simulink model "Online_Ordering_System_Component_Architecture"  (R2025a)
settings: Solver=VariableStepDiscrete  StartTime=0.0  StopTime=10.0  MaxStep=1  RelTol=1e-3
(part 1 of 2)
settings Model: Creator=OdaNobuyuki  LastModifiedBy=annic

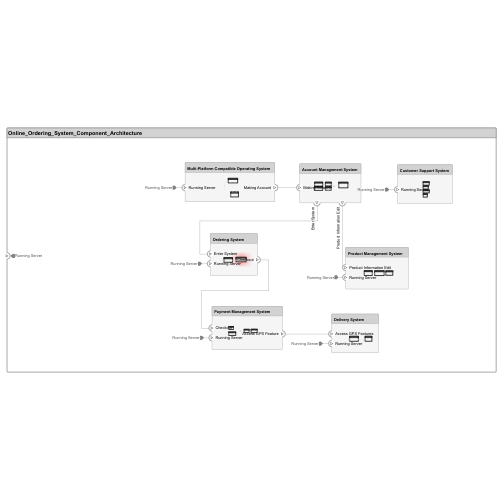
[thumbnail: Simulink's stored preview of the top-level diagram]
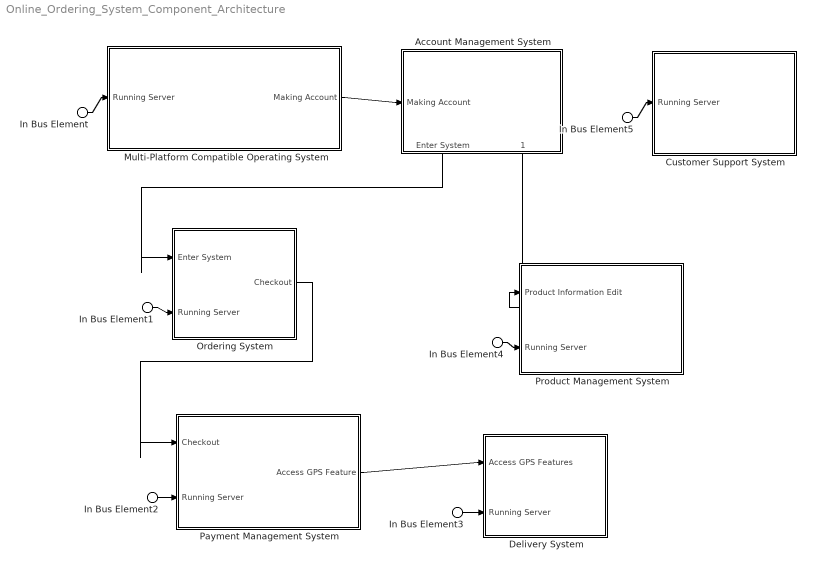
== system Online_Ordering_System_Component_Architecture ==
  In Bus Element{,1..5} (6 alike) : Inport  PortName=Running Server
  Account Management System : Subsystem
      settings: PortSchema="{\"entries\":[{\"content\":{\"headerSize\":26,\"margin\":15,\"minimumSpacing\":25,\"sides\":[{\"content\":{\"connectorIds\":[\"In1\"]},\"type\":\"ConnectorPlacement.EquallySpacedRectSide\",\"uuid\":\"d2ebed04-42f4-4bd6-aa56-c214d37abe86\"},{\"content\":{\"side\":\"RIGHT\"},\"type\":\"ConnectorPlacement.EquallySpacedRectSide\",\"uuid\":\"0a328130-2da5-4535-b8fd-dee261bd04a3\"},{\"content\":{\"side\":\"TOP\"},\"type\":\"ConnectorPlacement.EquallySpacedRectSide\",\"uuid\":\"410ea5eb-e20b-4523-bb7e-a86253749ceb\"},{\"content\":{\"connectorIds\":[\"Out2\",\"Out1\"],\"side\":\"BOTTOM\"},\"type\":\"ConnectorPlacement.EquallySpacedRectSide\",\"uuid\":\"972444bc-2579-4da8-b46a-55dab0c65c8e\"}]},\"type\":\"ConnectorPlacement.EquallySpacedConnector\",\"uuid\":\"5600d62f-d466-4629-981b-50f24b9b11a3\"}],\"packageUris\":[\"http://schema.mathworks.com/mf0/Connector/R2020b\"],\"version\":\"1.0\"}"
  "Customer Support System " : Subsystem
      settings: PortSchema="{\"entries\":[{\"content\":{\"headerSize\":26,\"margin\":15,\"minimumSpacing\":25,\"sides\":[{\"content\":{\"connectorIds\":[\"In1\"]},\"type\":\"ConnectorPlacement.EquallySpacedRectSide\",\"uuid\":\"fb288abb-f281-4c09-9d66-d398814e9f3f\"},{\"content\":{\"side\":\"RIGHT\"},\"type\":\"ConnectorPlacement.EquallySpacedRectSide\",\"uuid\":\"124df975-d2be-4c45-a02a-2f8c5952e2b0\"},{\"content\":{\"side\":\"TOP\"},\"type\":\"ConnectorPlacement.EquallySpacedRectSide\",\"uuid\":\"1b6fa379-ab8e-486c-bf17-64ebd19504fb\"}]},\"type\":\"ConnectorPlacement.EquallySpacedConnector\",\"uuid\":\"3496844b-ca8f-4528-b99e-6963a01fd8b6\"}],\"packageUris\":[\"http://schema.mathworks.com/mf0/Connector/R2020b\"],\"version\":\"1.0\"}"
  Delivery System : Subsystem
      settings: PortSchema="{\"entries\":[{\"content\":{\"headerSize\":26,\"margin\":15,\"minimumSpacing\":25,\"sides\":[{\"content\":{\"connectorIds\":[\"In1\",\"In2\"]},\"type\":\"ConnectorPlacement.EquallySpacedRectSide\",\"uuid\":\"d2ebed04-42f4-4bd6-aa56-c214d37abe86\"},{\"content\":{\"side\":\"RIGHT\"},\"type\":\"ConnectorPlacement.EquallySpacedRectSide\",\"uuid\":\"0a328130-2da5-4535-b8fd-dee261bd04a3\"},{\"content\":{\"side\":\"TOP\"},\"type\":\"ConnectorPlacement.EquallySpacedRectSide\",\"uuid\":\"410ea5eb-e20b-4523-bb7e-a86253749ceb\"}]},\"type\":\"ConnectorPlacement.EquallySpacedConnector\",\"uuid\":\"5600d62f-d466-4629-981b-50f24b9b11a3\"}],\"packageUris\":[\"http://schema.mathworks.com/mf0/Connector/R2020b\"],\"version\":\"1.0\"}"
  "Multi-Platform Compatible Operating System " : Subsystem
      settings: PortSchema="{\"entries\":[{\"content\":{\"headerSize\":26,\"margin\":15,\"minimumSpacing\":25,\"sides\":[{\"content\":{\"connectorIds\":[\"In1\"]},\"type\":\"ConnectorPlacement.EquallySpacedRectSide\",\"uuid\":\"fb288abb-f281-4c09-9d66-d398814e9f3f\"},{\"content\":{\"connectorIds\":[\"Out1\"],\"side\":\"RIGHT\"},\"type\":\"ConnectorPlacement.EquallySpacedRectSide\",\"uuid\":\"124df975-d2be-4c45-a02a-2f8c5952e2b0\"},{\"content\":{\"side\":\"TOP\"},\"type\":\"ConnectorPlacement.EquallySpacedRectSide\",\"uuid\":\"1b6fa379-ab8e-486c-bf17-64ebd19504fb\"}]},\"type\":\"ConnectorPlacement.EquallySpacedConnector\",\"uuid\":\"3496844b-ca8f-4528-b99e-6963a01fd8b6\"}],\"packageUris\":[\"http://schema.mathworks.com/mf0/Connector/R2020b\"],\"version\":\"1.0\"}"
  Ordering System : Subsystem
      settings: PortSchema="{\"entries\":[{\"content\":{\"headerSize\":26,\"margin\":15,\"minimumSpacing\":25,\"sides\":[{\"content\":{\"connectorIds\":[\"In1\",\"In2\"]},\"type\":\"ConnectorPlacement.EquallySpacedRectSide\",\"uuid\":\"fb288abb-f281-4c09-9d66-d398814e9f3f\"},{\"content\":{\"connectorIds\":[\"Out1\"],\"side\":\"RIGHT\"},\"type\":\"ConnectorPlacement.EquallySpacedRectSide\",\"uuid\":\"124df975-d2be-4c45-a02a-2f8c5952e2b0\"},{\"content\":{\"side\":\"TOP\"},\"type\":\"ConnectorPlacement.EquallySpacedRectSide\",\"uuid\":\"1b6fa379-ab8e-486c-bf17-64ebd19504fb\"}]},\"type\":\"ConnectorPlacement.EquallySpacedConnector\",\"uuid\":\"3496844b-ca8f-4528-b99e-6963a01fd8b6\"}],\"packageUris\":[\"http://schema.mathworks.com/mf0/Connector/R2020b\"],\"version\":\"1.0\"}"
  "Payment Management System " : Subsystem
      settings: PortSchema="{\"entries\":[{\"content\":{\"headerSize\":26,\"margin\":15,\"minimumSpacing\":25,\"sides\":[{\"content\":{\"connectorIds\":[\"In1\",\"In2\"]},\"type\":\"ConnectorPlacement.EquallySpacedRectSide\",\"uuid\":\"c87fdfc5-e8df-459e-b997-08543d0df41e\"},{\"content\":{\"connectorIds\":[\"Out1\"],\"side\":\"RIGHT\"},\"type\":\"ConnectorPlacement.EquallySpacedRectSide\",\"uuid\":\"2c60bf56-1d16-41c9-95da-6f31ce1e2453\"},{\"content\":{\"side\":\"TOP\"},\"type\":\"ConnectorPlacement.EquallySpacedRectSide\",\"uuid\":\"3204d3ae-6da8-4da9-829b-7d815393aaef\"}]},\"type\":\"ConnectorPlacement.EquallySpacedConnector\",\"uuid\":\"82e413f9-6f35-4bf6-9ebc-f322256f270e\"}],\"packageUris\":[\"http://schema.mathworks.com/mf0/Connector/R2020b\"],\"version\":\"1.0\"}"
  Product Management System : Subsystem
      settings: PortSchema="{\"entries\":[{\"content\":{\"headerSize\":26,\"margin\":15,\"minimumSpacing\":25,\"sides\":[{\"content\":{\"connectorIds\":[\"In1\",\"In2\"]},\"type\":\"ConnectorPlacement.EquallySpacedRectSide\",\"uuid\":\"fb288abb-f281-4c09-9d66-d398814e9f3f\"},{\"content\":{\"side\":\"RIGHT\"},\"type\":\"ConnectorPlacement.EquallySpacedRectSide\",\"uuid\":\"124df975-d2be-4c45-a02a-2f8c5952e2b0\"},{\"content\":{\"side\":\"TOP\"},\"type\":\"ConnectorPlacement.EquallySpacedRectSide\",\"uuid\":\"1b6fa379-ab8e-486c-bf17-64ebd19504fb\"}]},\"type\":\"ConnectorPlacement.EquallySpacedConnector\",\"uuid\":\"3496844b-ca8f-4528-b99e-6963a01fd8b6\"}],\"packageUris\":[\"http://schema.mathworks.com/mf0/Connector/R2020b\"],\"version\":\"1.0\"}"
  wires:
  In Bus Element/1 -> "Multi-Platform Compatible Operating System "/1(Running Server)
  In Bus Element1/1 -> Ordering System/2(Running Server)
  In Bus Element4/1 -> Product Management System/2(Running Server)
  In Bus Element5/1 -> "Customer Support System "/1(Running Server)
  Ordering System/1(Checkout) -> "Payment Management System "/1(Checkout)
  "Payment Management System "/1(Access GPS Feature) -> Delivery System/1(Access GPS Features)
  "Multi-Platform Compatible Operating System "/1(Making Account) -> Account Management System/1(Making Account)
  Account Management System/2(Enter System) -> Ordering System/1(Enter System)
  In Bus Element2/1 -> "Payment Management System "/2(Running Server)
  In Bus Element3/1 -> Delivery System/2(Running Server)
  Account Management System/1(Product Information Edit) -> Product Management System/1(Product Information Edit)

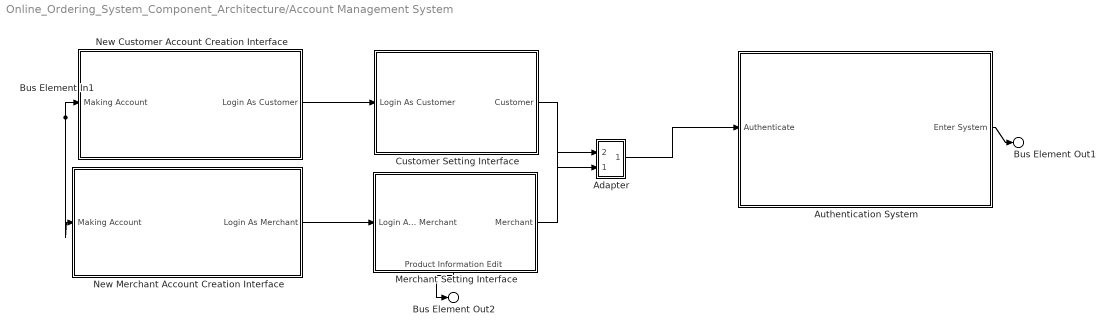
== system Online_Ordering_System_Component_Architecture/Account Management System ==
  Bus Element In1 : Inport  PortName=Making Account
  Adapter : Subsystem
      settings: PortSchema="{\"entries\":[{\"content\":{\"margin\":10,\"minimumSpacing\":15,\"sides\":[{\"content\":{\"connectorIds\":[\"In2\",\"In1\"]},\"type\":\"ConnectorPlacement.EquallySpacedRectSide\",\"uuid\":\"d2ebed04-42f4-4bd6-aa56-c214d37abe86\"},{\"content\":{\"connectorIds\":[\"Out1\"],\"side\":\"RIGHT\"},\"type\":\"ConnectorPlacement.EquallySpacedRectSide\",\"uuid\":\"0a328130-2da5-4535-b8fd-dee261bd04a3\"},{\"content\":{\"side\":\"TOP\"},\"type\":\"ConnectorPlacement.EquallySpacedRectSide\",\"uuid\":\"410ea5eb-e20b-4523-bb7e-a86253749ceb\"}]},\"type\":\"ConnectorPlacement.EquallySpacedConnector\",\"uuid\":\"5600d62f-d466-4629-981b-50f24b9b11a3\"}],\"packageUris\":[\"http://schema.mathworks.com/mf0/Connector/R2020b\"],\"version\":\"1.0\"}"
  "Authentication System " : Subsystem
      settings: PortSchema="{\"entries\":[{\"content\":{\"headerSize\":26,\"margin\":15,\"minimumSpacing\":25,\"sides\":[{\"content\":{\"connectorIds\":[\"In1\"]},\"type\":\"ConnectorPlacement.EquallySpacedRectSide\",\"uuid\":\"fb288abb-f281-4c09-9d66-d398814e9f3f\"},{\"content\":{\"connectorIds\":[\"Out1\"],\"side\":\"RIGHT\"},\"type\":\"ConnectorPlacement.EquallySpacedRectSide\",\"uuid\":\"124df975-d2be-4c45-a02a-2f8c5952e2b0\"},{\"content\":{\"side\":\"TOP\"},\"type\":\"ConnectorPlacement.EquallySpacedRectSide\",\"uuid\":\"1b6fa379-ab8e-486c-bf17-64ebd19504fb\"}]},\"type\":\"ConnectorPlacement.EquallySpacedConnector\",\"uuid\":\"3496844b-ca8f-4528-b99e-6963a01fd8b6\"}],\"packageUris\":[\"http://schema.mathworks.com/mf0/Connector/R2020b\"],\"version\":\"1.0\"}"
  Customer Setting Interface : Subsystem
      settings: PortSchema="{\"entries\":[{\"content\":{\"headerSize\":26,\"margin\":15,\"minimumSpacing\":25,\"sides\":[{\"content\":{\"connectorIds\":[\"In1\"]},\"type\":\"ConnectorPlacement.EquallySpacedRectSide\",\"uuid\":\"d2ebed04-42f4-4bd6-aa56-c214d37abe86\"},{\"content\":{\"connectorIds\":[\"Out1\"],\"side\":\"RIGHT\"},\"type\":\"ConnectorPlacement.EquallySpacedRectSide\",\"uuid\":\"0a328130-2da5-4535-b8fd-dee261bd04a3\"},{\"content\":{\"side\":\"TOP\"},\"type\":\"ConnectorPlacement.EquallySpacedRectSide\",\"uuid\":\"410ea5eb-e20b-4523-bb7e-a86253749ceb\"}]},\"type\":\"ConnectorPlacement.EquallySpacedConnector\",\"uuid\":\"5600d62f-d466-4629-981b-50f24b9b11a3\"}],\"packageUris\":[\"http://schema.mathworks.com/mf0/Connector/R2020b\"],\"version\":\"1.0\"}"
  Merchant Setting Interface : Subsystem
      settings: PortSchema="{\"entries\":[{\"content\":{\"headerSize\":26,\"margin\":15,\"minimumSpacing\":25,\"sides\":[{\"content\":{\"connectorIds\":[\"In1\"]},\"type\":\"ConnectorPlacement.EquallySpacedRectSide\",\"uuid\":\"d2ebed04-42f4-4bd6-aa56-c214d37abe86\"},{\"content\":{\"connectorIds\":[\"Out1\"],\"side\":\"RIGHT\"},\"type\":\"ConnectorPlacement.EquallySpacedRectSide\",\"uuid\":\"0a328130-2da5-4535-b8fd-dee261bd04a3\"},{\"content\":{\"side\":\"TOP\"},\"type\":\"ConnectorPlacement.EquallySpacedRectSide\",\"uuid\":\"410ea5eb-e20b-4523-bb7e-a86253749ceb\"},{\"content\":{\"connectorIds\":[\"Out2\"],\"side\":\"BOTTOM\"},\"type\":\"ConnectorPlacement.EquallySpacedRectSide\",\"uuid\":\"33d30d8b-b019-40dd-adb0-68cf80d802d6\"}]},\"type\":\"ConnectorPlacement.EquallySpacedConnector\",\"uuid\":\"5600d62f-d466-4629-981b-50f24b9b11a3\"}],\"packageUris\":[\"http://schema.mathworks.com/mf0/Connector/R2020b\"],\"version\":\"1.0\"}"
  New Customer Account Creation Interface : Subsystem
      settings: PortSchema="{\"entries\":[{\"content\":{\"headerSize\":26,\"margin\":15,\"minimumSpacing\":25,\"sides\":[{\"content\":{\"connectorIds\":[\"In1\"]},\"type\":\"ConnectorPlacement.EquallySpacedRectSide\",\"uuid\":\"d2ebed04-42f4-4bd6-aa56-c214d37abe86\"},{\"content\":{\"connectorIds\":[\"Out1\"],\"side\":\"RIGHT\"},\"type\":\"ConnectorPlacement.EquallySpacedRectSide\",\"uuid\":\"0a328130-2da5-4535-b8fd-dee261bd04a3\"},{\"content\":{\"side\":\"TOP\"},\"type\":\"ConnectorPlacement.EquallySpacedRectSide\",\"uuid\":\"410ea5eb-e20b-4523-bb7e-a86253749ceb\"}]},\"type\":\"ConnectorPlacement.EquallySpacedConnector\",\"uuid\":\"5600d62f-d466-4629-981b-50f24b9b11a3\"}],\"packageUris\":[\"http://schema.mathworks.com/mf0/Connector/R2020b\"],\"version\":\"1.0\"}"
  New Merchant Account Creation Interface : Subsystem
      settings: PortSchema="{\"entries\":[{\"content\":{\"headerSize\":26,\"margin\":15,\"minimumSpacing\":25,\"sides\":[{\"content\":{\"connectorIds\":[\"In1\"]},\"type\":\"ConnectorPlacement.EquallySpacedRectSide\",\"uuid\":\"d2ebed04-42f4-4bd6-aa56-c214d37abe86\"},{\"content\":{\"connectorIds\":[\"Out1\"],\"side\":\"RIGHT\"},\"type\":\"ConnectorPlacement.EquallySpacedRectSide\",\"uuid\":\"0a328130-2da5-4535-b8fd-dee261bd04a3\"},{\"content\":{\"side\":\"TOP\"},\"type\":\"ConnectorPlacement.EquallySpacedRectSide\",\"uuid\":\"410ea5eb-e20b-4523-bb7e-a86253749ceb\"},{\"content\":{\"side\":\"BOTTOM\"},\"type\":\"ConnectorPlacement.EquallySpacedRectSide\",\"uuid\":\"ea88bfd1-3edf-4a24-905e-339c6eca56ba\"}]},\"type\":\"ConnectorPlacement.EquallySpacedConnector\",\"uuid\":\"5600d62f-d466-4629-981b-50f24b9b11a3\"}],\"packageUris\":[\"http://schema.mathworks.com/mf0/Connector/R2020b\"],\"version\":\"1.0\"}"
  Bus Element Out2 : Outport  PortName=Product Information Edit
  Bus Element Out1 : Outport  Port=2  PortName=Enter System
  wires:
  New Customer Account Creation Interface/1(Login As Customer) -> Customer Setting Interface/1(Login As Customer)
  New Merchant Account Creation Interface/1(Login As Merchant) -> Merchant Setting Interface/1(Login As Merchant)
  "Authentication System "/1(Enter System) -> Bus Element Out1/1
  Bus Element In1/1 -> New Merchant Account Creation Interface/1(Making Account), New Customer Account Creation Interface/1(Making Account)
  Customer Setting Interface/1(Customer) -> Adapter/2(Customer)
  Merchant Setting Interface/2(Product Information Edit) -> Bus Element Out2/1
  Merchant Setting Interface/1(Merchant) -> Adapter/1(Merchant)
  Adapter/1(Authenticate) -> "Authentication System "/1(Authenticate)

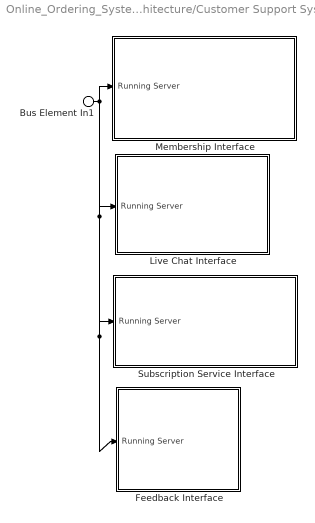
== system Online_Ordering_System_Component_Architecture/Customer Support System  ==
  Bus Element In1 : Inport  PortName=Running Server
  Feedback Interface : Subsystem
      settings: PortSchema="{\"entries\":[{\"content\":{\"headerSize\":26,\"margin\":15,\"minimumSpacing\":25,\"sides\":[{\"content\":{\"connectorIds\":[\"In1\"]},\"type\":\"ConnectorPlacement.EquallySpacedRectSide\",\"uuid\":\"c87fdfc5-e8df-459e-b997-08543d0df41e\"},{\"content\":{\"side\":\"RIGHT\"},\"type\":\"ConnectorPlacement.EquallySpacedRectSide\",\"uuid\":\"2c60bf56-1d16-41c9-95da-6f31ce1e2453\"},{\"content\":{\"side\":\"TOP\"},\"type\":\"ConnectorPlacement.EquallySpacedRectSide\",\"uuid\":\"3204d3ae-6da8-4da9-829b-7d815393aaef\"},{\"content\":{\"side\":\"BOTTOM\"},\"type\":\"ConnectorPlacement.EquallySpacedRectSide\",\"uuid\":\"977d6b67-58e6-4ded-b369-a817140b3543\"}]},\"type\":\"ConnectorPlacement.EquallySpacedConnector\",\"uuid\":\"82e413f9-6f35-4bf6-9ebc-f322256f270e\"}],\"packageUris\":[\"http://schema.mathworks.com/mf0/Connector/R2020b\"],\"version\":\"1.0\"}"
  Live Chat Interface : Subsystem
      settings: PortSchema="{\"entries\":[{\"content\":{\"headerSize\":26,\"margin\":15,\"minimumSpacing\":25,\"sides\":[{\"content\":{\"connectorIds\":[\"In1\"]},\"type\":\"ConnectorPlacement.EquallySpacedRectSide\",\"uuid\":\"c87fdfc5-e8df-459e-b997-08543d0df41e\"},{\"content\":{\"side\":\"RIGHT\"},\"type\":\"ConnectorPlacement.EquallySpacedRectSide\",\"uuid\":\"2c60bf56-1d16-41c9-95da-6f31ce1e2453\"},{\"content\":{\"side\":\"TOP\"},\"type\":\"ConnectorPlacement.EquallySpacedRectSide\",\"uuid\":\"3204d3ae-6da8-4da9-829b-7d815393aaef\"}]},\"type\":\"ConnectorPlacement.EquallySpacedConnector\",\"uuid\":\"82e413f9-6f35-4bf6-9ebc-f322256f270e\"}],\"packageUris\":[\"http://schema.mathworks.com/mf0/Connector/R2020b\"],\"version\":\"1.0\"}"
  Membership Interface : Subsystem
      settings: PortSchema="{\"entries\":[{\"content\":{\"headerSize\":26,\"margin\":15,\"minimumSpacing\":25,\"sides\":[{\"content\":{\"connectorIds\":[\"In1\"]},\"type\":\"ConnectorPlacement.EquallySpacedRectSide\",\"uuid\":\"c87fdfc5-e8df-459e-b997-08543d0df41e\"},{\"content\":{\"side\":\"RIGHT\"},\"type\":\"ConnectorPlacement.EquallySpacedRectSide\",\"uuid\":\"2c60bf56-1d16-41c9-95da-6f31ce1e2453\"},{\"content\":{\"side\":\"TOP\"},\"type\":\"ConnectorPlacement.EquallySpacedRectSide\",\"uuid\":\"3204d3ae-6da8-4da9-829b-7d815393aaef\"}]},\"type\":\"ConnectorPlacement.EquallySpacedConnector\",\"uuid\":\"82e413f9-6f35-4bf6-9ebc-f322256f270e\"}],\"packageUris\":[\"http://schema.mathworks.com/mf0/Connector/R2020b\"],\"version\":\"1.0\"}"
  Subscription Service Interface : Subsystem
      settings: PortSchema="{\"entries\":[{\"content\":{\"headerSize\":26,\"margin\":15,\"minimumSpacing\":25,\"sides\":[{\"content\":{\"connectorIds\":[\"In1\"]},\"type\":\"ConnectorPlacement.EquallySpacedRectSide\",\"uuid\":\"c87fdfc5-e8df-459e-b997-08543d0df41e\"},{\"content\":{\"side\":\"RIGHT\"},\"type\":\"ConnectorPlacement.EquallySpacedRectSide\",\"uuid\":\"2c60bf56-1d16-41c9-95da-6f31ce1e2453\"},{\"content\":{\"side\":\"TOP\"},\"type\":\"ConnectorPlacement.EquallySpacedRectSide\",\"uuid\":\"3204d3ae-6da8-4da9-829b-7d815393aaef\"}]},\"type\":\"ConnectorPlacement.EquallySpacedConnector\",\"uuid\":\"82e413f9-6f35-4bf6-9ebc-f322256f270e\"}],\"packageUris\":[\"http://schema.mathworks.com/mf0/Connector/R2020b\"],\"version\":\"1.0\"}"
  wires:
  Bus Element In1/1 -> Feedback Interface/1(Running Server), Subscription Service Interface/1(Running Server), Live Chat Interface/1(Running Server), Membership Interface/1(Running Server)

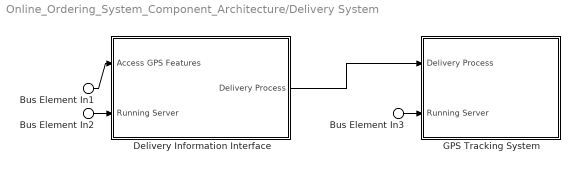
== system Online_Ordering_System_Component_Architecture/Delivery System ==
  Bus Element In1 : Inport  PortName=Access GPS Features
  Bus Element In2 : Inport  Port=2  PortName=Running Server
  Bus Element In3 : Inport  Port=2  PortName=Running Server
  Delivery Information Interface : Subsystem
      settings: PortSchema="{\"entries\":[{\"content\":{\"headerSize\":26,\"margin\":15,\"minimumSpacing\":25,\"sides\":[{\"content\":{\"connectorIds\":[\"In1\",\"In2\"]},\"type\":\"ConnectorPlacement.EquallySpacedRectSide\",\"uuid\":\"d2ebed04-42f4-4bd6-aa56-c214d37abe86\"},{\"content\":{\"connectorIds\":[\"Out1\"],\"side\":\"RIGHT\"},\"type\":\"ConnectorPlacement.EquallySpacedRectSide\",\"uuid\":\"0a328130-2da5-4535-b8fd-dee261bd04a3\"},{\"content\":{\"side\":\"TOP\"},\"type\":\"ConnectorPlacement.EquallySpacedRectSide\",\"uuid\":\"410ea5eb-e20b-4523-bb7e-a86253749ceb\"}]},\"type\":\"ConnectorPlacement.EquallySpacedConnector\",\"uuid\":\"5600d62f-d466-4629-981b-50f24b9b11a3\"}],\"packageUris\":[\"http://schema.mathworks.com/mf0/Connector/R2020b\"],\"version\":\"1.0\"}"
  GPS Tracking System : Subsystem
      settings: PortSchema="{\"entries\":[{\"content\":{\"headerSize\":26,\"margin\":15,\"minimumSpacing\":25,\"sides\":[{\"content\":{\"connectorIds\":[\"In1\",\"In2\"]},\"type\":\"ConnectorPlacement.EquallySpacedRectSide\",\"uuid\":\"d2ebed04-42f4-4bd6-aa56-c214d37abe86\"},{\"content\":{\"side\":\"RIGHT\"},\"type\":\"ConnectorPlacement.EquallySpacedRectSide\",\"uuid\":\"0a328130-2da5-4535-b8fd-dee261bd04a3\"},{\"content\":{\"side\":\"TOP\"},\"type\":\"ConnectorPlacement.EquallySpacedRectSide\",\"uuid\":\"410ea5eb-e20b-4523-bb7e-a86253749ceb\"}]},\"type\":\"ConnectorPlacement.EquallySpacedConnector\",\"uuid\":\"5600d62f-d466-4629-981b-50f24b9b11a3\"}],\"packageUris\":[\"http://schema.mathworks.com/mf0/Connector/R2020b\"],\"version\":\"1.0\"}"
  wires:
  Delivery Information Interface/1(Delivery Process) -> GPS Tracking System/1(Delivery Process)
  Bus Element In1/1 -> Delivery Information Interface/1(Access GPS Features)
  Bus Element In2/1 -> Delivery Information Interface/2(Running Server)
  Bus Element In3/1 -> GPS Tracking System/2(Running Server)

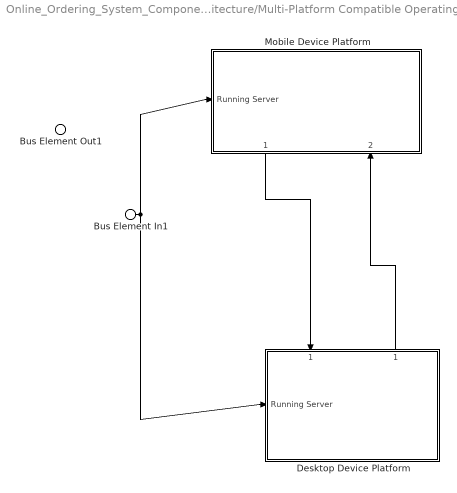
== system Online_Ordering_System_Component_Architecture/Multi-Platform Compatible Operating System  ==
  Bus Element In1 : Inport  PortName=Running Server
  Desktop Device Platform : Subsystem
      settings: PortSchema="{\"entries\":[{\"content\":{\"headerSize\":26,\"margin\":15,\"minimumSpacing\":25,\"sides\":[{\"content\":{\"connectorIds\":[\"In2\"]},\"type\":\"ConnectorPlacement.EquallySpacedRectSide\",\"uuid\":\"c87fdfc5-e8df-459e-b997-08543d0df41e\"},{\"content\":{\"side\":\"RIGHT\"},\"type\":\"ConnectorPlacement.EquallySpacedRectSide\",\"uuid\":\"2c60bf56-1d16-41c9-95da-6f31ce1e2453\"},{\"content\":{\"connectorIds\":[\"In1\",\"Out1\"],\"side\":\"TOP\"},\"type\":\"ConnectorPlacement.EquallySpacedRectSide\",\"uuid\":\"3204d3ae-6da8-4da9-829b-7d815393aaef\"}]},\"type\":\"ConnectorPlacement.EquallySpacedConnector\",\"uuid\":\"82e413f9-6f35-4bf6-9ebc-f322256f270e\"}],\"packageUris\":[\"http://schema.mathworks.com/mf0/Connector/R2020b\"],\"version\":\"1.0\"}"
  Mobile Device Platform : Subsystem
      settings: PortSchema="{\"entries\":[{\"content\":{\"headerSize\":26,\"margin\":15,\"minimumSpacing\":25,\"sides\":[{\"content\":{\"connectorIds\":[\"In1\"]},\"type\":\"ConnectorPlacement.EquallySpacedRectSide\",\"uuid\":\"c87fdfc5-e8df-459e-b997-08543d0df41e\"},{\"content\":{\"side\":\"RIGHT\"},\"type\":\"ConnectorPlacement.EquallySpacedRectSide\",\"uuid\":\"2c60bf56-1d16-41c9-95da-6f31ce1e2453\"},{\"content\":{\"side\":\"TOP\"},\"type\":\"ConnectorPlacement.EquallySpacedRectSide\",\"uuid\":\"3204d3ae-6da8-4da9-829b-7d815393aaef\"},{\"content\":{\"connectorIds\":[\"Out1\",\"In2\"],\"side\":\"BOTTOM\"},\"type\":\"ConnectorPlacement.EquallySpacedRectSide\",\"uuid\":\"10b8ba8c-a9af-4eed-8b19-4e9933e8a974\"}]},\"type\":\"ConnectorPlacement.EquallySpacedConnector\",\"uuid\":\"82e413f9-6f35-4bf6-9ebc-f322256f270e\"}],\"packageUris\":[\"http://schema.mathworks.com/mf0/Connector/R2020b\"],\"version\":\"1.0\"}"
  Bus Element Out1 : Outport  PortName=Making Account
  wires:
  Mobile Device Platform/1(Data Share From Mobile Devices) -> Desktop Device Platform/1(Data Share From Mobile Devices)
  Desktop Device Platform/1(Data Share From PC / Laptop) -> Mobile Device Platform/2(Data Share From PC / Laptop)
  Bus Element In1/1 -> Desktop Device Platform/2(Running Server), Mobile Device Platform/1(Running Server)

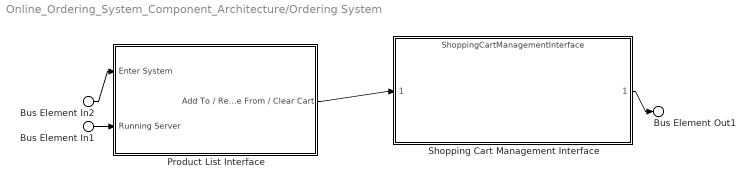
== system Online_Ordering_System_Component_Architecture/Ordering System ==
  Bus Element In2 : Inport  PortName=Enter System
  Bus Element In1 : Inport  Port=2  PortName=Running Server
  Product List Interface : Subsystem
      settings: PortSchema="{\"entries\":[{\"content\":{\"headerSize\":26,\"margin\":15,\"minimumSpacing\":25,\"sides\":[{\"content\":{\"connectorIds\":[\"In1\",\"In2\"]},\"type\":\"ConnectorPlacement.EquallySpacedRectSide\",\"uuid\":\"c87fdfc5-e8df-459e-b997-08543d0df41e\"},{\"content\":{\"connectorIds\":[\"Out1\"],\"side\":\"RIGHT\"},\"type\":\"ConnectorPlacement.EquallySpacedRectSide\",\"uuid\":\"2c60bf56-1d16-41c9-95da-6f31ce1e2453\"},{\"content\":{\"side\":\"TOP\"},\"type\":\"ConnectorPlacement.EquallySpacedRectSide\",\"uuid\":\"3204d3ae-6da8-4da9-829b-7d815393aaef\"}]},\"type\":\"ConnectorPlacement.EquallySpacedConnector\",\"uuid\":\"82e413f9-6f35-4bf6-9ebc-f322256f270e\"}],\"packageUris\":[\"http://schema.mathworks.com/mf0/Connector/R2020b\"],\"version\":\"1.0\"}"
  Shopping Cart Management Interface : ModelReference  ModelNameDialog=ShoppingCartManagementInterface  SimulationMode=Normal  ModelReferenceVersion=1.11
      settings: PortSchema="{\"entries\":[{\"content\":{\"headerSize\":38,\"margin\":15,\"minimumSpacing\":25,\"sides\":[{\"content\":{\"connectorIds\":[\"In1\"]},\"type\":\"ConnectorPlacement.EquallySpacedRectSide\",\"uuid\":\"d2ebed04-42f4-4bd6-aa56-c214d37abe86\"},{\"content\":{\"connectorIds\":[\"Out1\"],\"side\":\"RIGHT\"},\"type\":\"ConnectorPlacement.EquallySpacedRectSide\",\"uuid\":\"0a328130-2da5-4535-b8fd-dee261bd04a3\"},{\"content\":{\"side\":\"TOP\"},\"type\":\"ConnectorPlacement.EquallySpacedRectSide\",\"uuid\":\"410ea5eb-e20b-4523-bb7e-a86253749ceb\"}]},\"type\":\"ConnectorPlacement.EquallySpacedConnector\",\"uuid\":\"5600d62f-d466-4629-981b-50f24b9b11a3\"}],\"packageUris\":[\"http://schema.mathworks.com/mf0/Connector/R2020b\"],\"version\":\"1.0\"}"
  Bus Element Out1 : Outport  PortName=Checkout
  wires:
  Bus Element In2/1 -> Product List Interface/1(Enter System)
  Bus Element In1/1 -> Product List Interface/2(Running Server)
  Product List Interface/1(Add To / Remove From / Clear Cart) -> Shopping Cart Management Interface/1
  Shopping Cart Management Interface/1 -> Bus Element Out1/1

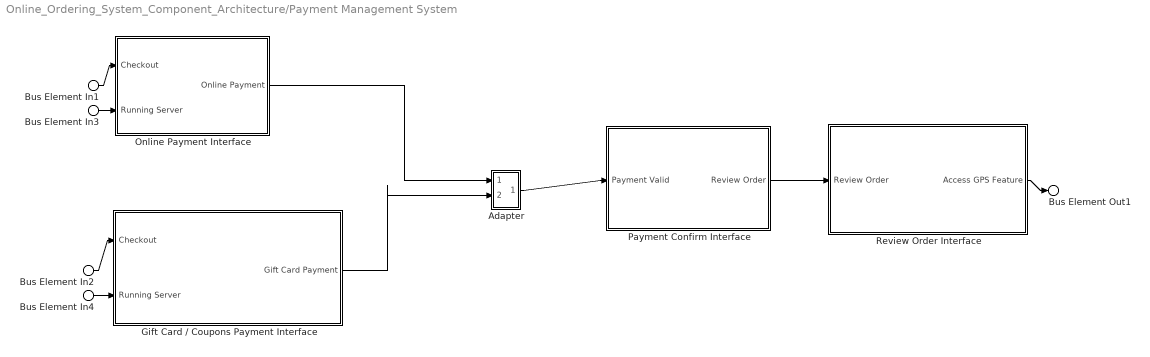
== system Online_Ordering_System_Component_Architecture/Payment Management System  ==
  Bus Element In1 : Inport  PortName=Checkout
  Bus Element In2 : Inport  PortName=Checkout
  Bus Element In3 : Inport  Port=2  PortName=Running Server
  Bus Element In4 : Inport  Port=2  PortName=Running Server
  " Gift Card / Coupons Payment Interface" : Subsystem
      settings: PortSchema="{\"entries\":[{\"content\":{\"headerSize\":26,\"margin\":15,\"minimumSpacing\":25,\"sides\":[{\"content\":{\"connectorIds\":[\"In1\",\"In2\"]},\"type\":\"ConnectorPlacement.EquallySpacedRectSide\",\"uuid\":\"c87fdfc5-e8df-459e-b997-08543d0df41e\"},{\"content\":{\"connectorIds\":[\"Out1\"],\"side\":\"RIGHT\"},\"type\":\"ConnectorPlacement.EquallySpacedRectSide\",\"uuid\":\"2c60bf56-1d16-41c9-95da-6f31ce1e2453\"},{\"content\":{\"side\":\"TOP\"},\"type\":\"ConnectorPlacement.EquallySpacedRectSide\",\"uuid\":\"3204d3ae-6da8-4da9-829b-7d815393aaef\"}]},\"type\":\"ConnectorPlacement.EquallySpacedConnector\",\"uuid\":\"82e413f9-6f35-4bf6-9ebc-f322256f270e\"}],\"packageUris\":[\"http://schema.mathworks.com/mf0/Connector/R2020b\"],\"version\":\"1.0\"}"
  Adapter : Subsystem
      settings: PortSchema="{\"entries\":[{\"content\":{\"margin\":10,\"minimumSpacing\":15,\"sides\":[{\"content\":{\"connectorIds\":[\"In1\",\"In2\"]},\"type\":\"ConnectorPlacement.EquallySpacedRectSide\",\"uuid\":\"d2ebed04-42f4-4bd6-aa56-c214d37abe86\"},{\"content\":{\"connectorIds\":[\"Out1\"],\"side\":\"RIGHT\"},\"type\":\"ConnectorPlacement.EquallySpacedRectSide\",\"uuid\":\"0a328130-2da5-4535-b8fd-dee261bd04a3\"},{\"content\":{\"side\":\"TOP\"},\"type\":\"ConnectorPlacement.EquallySpacedRectSide\",\"uuid\":\"410ea5eb-e20b-4523-bb7e-a86253749ceb\"}]},\"type\":\"ConnectorPlacement.EquallySpacedConnector\",\"uuid\":\"5600d62f-d466-4629-981b-50f24b9b11a3\"}],\"packageUris\":[\"http://schema.mathworks.com/mf0/Connector/R2020b\"],\"version\":\"1.0\"}"
  Online Payment Interface : Subsystem
      settings: PortSchema="{\"entries\":[{\"content\":{\"headerSize\":26,\"margin\":15,\"minimumSpacing\":25,\"sides\":[{\"content\":{\"connectorIds\":[\"In1\",\"In2\"]},\"type\":\"ConnectorPlacement.EquallySpacedRectSide\",\"uuid\":\"c87fdfc5-e8df-459e-b997-08543d0df41e\"},{\"content\":{\"connectorIds\":[\"Out1\"],\"side\":\"RIGHT\"},\"type\":\"ConnectorPlacement.EquallySpacedRectSide\",\"uuid\":\"2c60bf56-1d16-41c9-95da-6f31ce1e2453\"},{\"content\":{\"side\":\"TOP\"},\"type\":\"ConnectorPlacement.EquallySpacedRectSide\",\"uuid\":\"3204d3ae-6da8-4da9-829b-7d815393aaef\"}]},\"type\":\"ConnectorPlacement.EquallySpacedConnector\",\"uuid\":\"82e413f9-6f35-4bf6-9ebc-f322256f270e\"}],\"packageUris\":[\"http://schema.mathworks.com/mf0/Connector/R2020b\"],\"version\":\"1.0\"}"
  Payment Confirm Interface : Subsystem
      settings: PortSchema="{\"entries\":[{\"content\":{\"headerSize\":26,\"margin\":15,\"minimumSpacing\":25,\"sides\":[{\"content\":{\"connectorIds\":[\"In1\"]},\"type\":\"ConnectorPlacement.EquallySpacedRectSide\",\"uuid\":\"d2ebed04-42f4-4bd6-aa56-c214d37abe86\"},{\"content\":{\"connectorIds\":[\"Out1\"],\"side\":\"RIGHT\"},\"type\":\"ConnectorPlacement.EquallySpacedRectSide\",\"uuid\":\"0a328130-2da5-4535-b8fd-dee261bd04a3\"},{\"content\":{\"side\":\"TOP\"},\"type\":\"ConnectorPlacement.EquallySpacedRectSide\",\"uuid\":\"410ea5eb-e20b-4523-bb7e-a86253749ceb\"}]},\"type\":\"ConnectorPlacement.EquallySpacedConnector\",\"uuid\":\"5600d62f-d466-4629-981b-50f24b9b11a3\"}],\"packageUris\":[\"http://schema.mathworks.com/mf0/Connector/R2020b\"],\"version\":\"1.0\"}"
  Review Order Interface : Subsystem
      settings: PortSchema="{\"entries\":[{\"content\":{\"headerSize\":26,\"margin\":15,\"minimumSpacing\":25,\"sides\":[{\"content\":{\"connectorIds\":[\"In1\"]},\"type\":\"ConnectorPlacement.EquallySpacedRectSide\",\"uuid\":\"d2ebed04-42f4-4bd6-aa56-c214d37abe86\"},{\"content\":{\"connectorIds\":[\"Out1\"],\"side\":\"RIGHT\"},\"type\":\"ConnectorPlacement.EquallySpacedRectSide\",\"uuid\":\"0a328130-2da5-4535-b8fd-dee261bd04a3\"},{\"content\":{\"side\":\"TOP\"},\"type\":\"ConnectorPlacement.EquallySpacedRectSide\",\"uuid\":\"410ea5eb-e20b-4523-bb7e-a86253749ceb\"}]},\"type\":\"ConnectorPlacement.EquallySpacedConnector\",\"uuid\":\"5600d62f-d466-4629-981b-50f24b9b11a3\"}],\"packageUris\":[\"http://schema.mathworks.com/mf0/Connector/R2020b\"],\"version\":\"1.0\"}"
  Bus Element Out1 : Outport  PortName=Access GPS Feature
  wires:
  Bus Element In1/1 -> Online Payment Interface/1(Checkout)
  Bus Element In2/1 -> " Gift Card / Coupons Payment Interface"/1(Checkout)
  Online Payment Interface/1(Online Payment) -> Adapter/1(Online Payment)
  " Gift Card / Coupons Payment Interface"/1(Gift Card Payment) -> Adapter/2(Gift Card Payment)
  Adapter/1(Payment Valid) -> Payment Confirm Interface/1(Payment Valid)
  Payment Confirm Interface/1(Review Order) -> Review Order Interface/1(Review Order)
  Review Order Interface/1(Access GPS Feature) -> Bus Element Out1/1
  Bus Element In3/1 -> Online Payment Interface/2(Running Server)
  Bus Element In4/1 -> " Gift Card / Coupons Payment Interface"/2(Running Server)

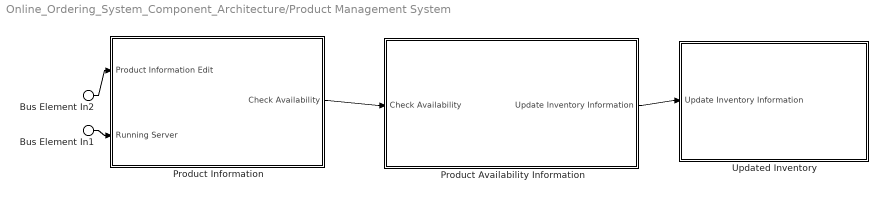
== system Online_Ordering_System_Component_Architecture/Product Management System ==
  Bus Element In2 : Inport  PortName=Product Information Edit
  Bus Element In1 : Inport  Port=2  PortName=Running Server
  Product Availability Information : Subsystem
      settings: PortSchema="{\"entries\":[{\"content\":{\"headerSize\":26,\"margin\":15,\"minimumSpacing\":25,\"sides\":[{\"content\":{\"connectorIds\":[\"In1\"]},\"type\":\"ConnectorPlacement.EquallySpacedRectSide\",\"uuid\":\"d2ebed04-42f4-4bd6-aa56-c214d37abe86\"},{\"content\":{\"connectorIds\":[\"Out1\"],\"side\":\"RIGHT\"},\"type\":\"ConnectorPlacement.EquallySpacedRectSide\",\"uuid\":\"0a328130-2da5-4535-b8fd-dee261bd04a3\"},{\"content\":{\"side\":\"TOP\"},\"type\":\"ConnectorPlacement.EquallySpacedRectSide\",\"uuid\":\"410ea5eb-e20b-4523-bb7e-a86253749ceb\"},{\"content\":{\"side\":\"BOTTOM\"},\"type\":\"ConnectorPlacement.EquallySpacedRectSide\",\"uuid\":\"93bf66a0-1f21-442e-9174-313184729b7c\"}]},\"type\":\"ConnectorPlacement.EquallySpacedConnector\",\"uuid\":\"5600d62f-d466-4629-981b-50f24b9b11a3\"}],\"packageUris\":[\"http://schema.mathworks.com/mf0/Connector/R2020b\"],\"version\":\"1.0\"}"
  Product Information : Subsystem
      settings: PortSchema="{\"entries\":[{\"content\":{\"headerSize\":26,\"margin\":15,\"minimumSpacing\":25,\"sides\":[{\"content\":{\"connectorIds\":[\"In1\",\"In2\"]},\"type\":\"ConnectorPlacement.EquallySpacedRectSide\",\"uuid\":\"d2ebed04-42f4-4bd6-aa56-c214d37abe86\"},{\"content\":{\"connectorIds\":[\"Out1\"],\"side\":\"RIGHT\"},\"type\":\"ConnectorPlacement.EquallySpacedRectSide\",\"uuid\":\"0a328130-2da5-4535-b8fd-dee261bd04a3\"},{\"content\":{\"side\":\"TOP\"},\"type\":\"ConnectorPlacement.EquallySpacedRectSide\",\"uuid\":\"410ea5eb-e20b-4523-bb7e-a86253749ceb\"},{\"content\":{\"side\":\"BOTTOM\"},\"type\":\"ConnectorPlacement.EquallySpacedRectSide\",\"uuid\":\"726e7944-675c-4839-b437-a1bae54df8ca\"}]},\"type\":\"ConnectorPlacement.EquallySpacedConnector\",\"uuid\":\"5600d62f-d466-4629-981b-50f24b9b11a3\"}],\"packageUris\":[\"http://schema.mathworks.com/mf0/Connector/R2020b\"],\"version\":\"1.0\"}"
  Updated Inventory : Subsystem
      settings: PortSchema="{\"entries\":[{\"content\":{\"headerSize\":26,\"margin\":15,\"minimumSpacing\":25,\"sides\":[{\"content\":{\"connectorIds\":[\"In1\"]},\"type\":\"ConnectorPlacement.EquallySpacedRectSide\",\"uuid\":\"d2ebed04-42f4-4bd6-aa56-c214d37abe86\"},{\"content\":{\"side\":\"RIGHT\"},\"type\":\"ConnectorPlacement.EquallySpacedRectSide\",\"uuid\":\"0a328130-2da5-4535-b8fd-dee261bd04a3\"},{\"content\":{\"side\":\"TOP\"},\"type\":\"ConnectorPlacement.EquallySpacedRectSide\",\"uuid\":\"410ea5eb-e20b-4523-bb7e-a86253749ceb\"}]},\"type\":\"ConnectorPlacement.EquallySpacedConnector\",\"uuid\":\"5600d62f-d466-4629-981b-50f24b9b11a3\"}],\"packageUris\":[\"http://schema.mathworks.com/mf0/Connector/R2020b\"],\"version\":\"1.0\"}"
  wires:
  Product Information/1(Check Availability) -> Product Availability Information/1(Check Availability)
  Product Availability Information/1(Update Inventory Information) -> Updated Inventory/1(Update Inventory Information)
  Bus Element In2/1 -> Product Information/1(Product Information Edit)
  Bus Element In1/1 -> Product Information/2(Running Server)

== system Online_Ordering_System_Component_Architecture/Account Management System/Adapter ==
  Bus Element In1 : Inport  PortName=Merchant
  In Bus Element : Inport  Port=2  PortName=Customer
  Out Bus Element : Outport  PortName=Authenticate
  wires:
  In Bus Element/1 -> Out Bus Element/1

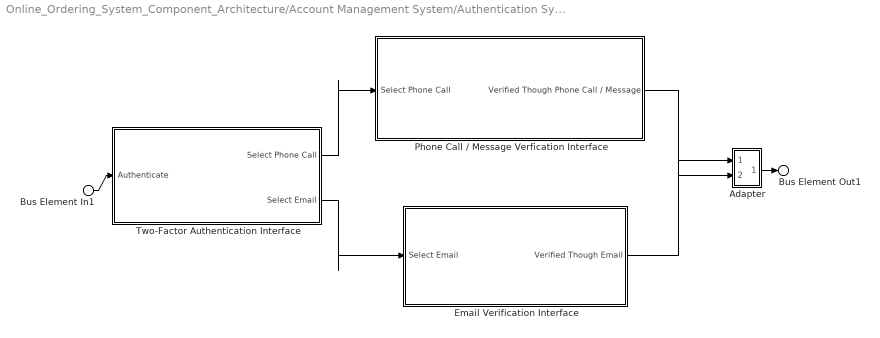
== system Online_Ordering_System_Component_Architecture/Account Management System/Authentication System  ==
  Bus Element In1 : Inport  PortName=Authenticate
  Adapter : Subsystem
      settings: PortSchema="{\"entries\":[{\"content\":{\"margin\":10,\"minimumSpacing\":15,\"sides\":[{\"content\":{\"connectorIds\":[\"In1\",\"In2\"]},\"type\":\"ConnectorPlacement.EquallySpacedRectSide\",\"uuid\":\"c87fdfc5-e8df-459e-b997-08543d0df41e\"},{\"content\":{\"connectorIds\":[\"Out1\"],\"side\":\"RIGHT\"},\"type\":\"ConnectorPlacement.EquallySpacedRectSide\",\"uuid\":\"2c60bf56-1d16-41c9-95da-6f31ce1e2453\"},{\"content\":{\"side\":\"TOP\"},\"type\":\"ConnectorPlacement.EquallySpacedRectSide\",\"uuid\":\"3204d3ae-6da8-4da9-829b-7d815393aaef\"}]},\"type\":\"ConnectorPlacement.EquallySpacedConnector\",\"uuid\":\"82e413f9-6f35-4bf6-9ebc-f322256f270e\"}],\"packageUris\":[\"http://schema.mathworks.com/mf0/Connector/R2020b\"],\"version\":\"1.0\"}"
  Email Verification Interface : Subsystem
      settings: PortSchema="{\"entries\":[{\"content\":{\"headerSize\":26,\"margin\":15,\"minimumSpacing\":25,\"sides\":[{\"content\":{\"connectorIds\":[\"In1\"]},\"type\":\"ConnectorPlacement.EquallySpacedRectSide\",\"uuid\":\"c87fdfc5-e8df-459e-b997-08543d0df41e\"},{\"content\":{\"connectorIds\":[\"Out1\"],\"side\":\"RIGHT\"},\"type\":\"ConnectorPlacement.EquallySpacedRectSide\",\"uuid\":\"2c60bf56-1d16-41c9-95da-6f31ce1e2453\"},{\"content\":{\"side\":\"TOP\"},\"type\":\"ConnectorPlacement.EquallySpacedRectSide\",\"uuid\":\"3204d3ae-6da8-4da9-829b-7d815393aaef\"}]},\"type\":\"ConnectorPlacement.EquallySpacedConnector\",\"uuid\":\"82e413f9-6f35-4bf6-9ebc-f322256f270e\"}],\"packageUris\":[\"http://schema.mathworks.com/mf0/Connector/R2020b\"],\"version\":\"1.0\"}"
  Phone Call / Message Verfication Interface : Subsystem
      settings: PortSchema="{\"entries\":[{\"content\":{\"headerSize\":26,\"margin\":15,\"minimumSpacing\":25,\"sides\":[{\"content\":{\"connectorIds\":[\"In1\"]},\"type\":\"ConnectorPlacement.EquallySpacedRectSide\",\"uuid\":\"c87fdfc5-e8df-459e-b997-08543d0df41e\"},{\"content\":{\"connectorIds\":[\"Out1\"],\"side\":\"RIGHT\"},\"type\":\"ConnectorPlacement.EquallySpacedRectSide\",\"uuid\":\"2c60bf56-1d16-41c9-95da-6f31ce1e2453\"},{\"content\":{\"side\":\"TOP\"},\"type\":\"ConnectorPlacement.EquallySpacedRectSide\",\"uuid\":\"3204d3ae-6da8-4da9-829b-7d815393aaef\"}]},\"type\":\"ConnectorPlacement.EquallySpacedConnector\",\"uuid\":\"82e413f9-6f35-4bf6-9ebc-f322256f270e\"}],\"packageUris\":[\"http://schema.mathworks.com/mf0/Connector/R2020b\"],\"version\":\"1.0\"}"
  Two-Factor Authentication Interface : Subsystem
      settings: PortSchema="{\"entries\":[{\"content\":{\"headerSize\":26,\"margin\":15,\"minimumSpacing\":25,\"sides\":[{\"content\":{\"connectorIds\":[\"In1\"]},\"type\":\"ConnectorPlacement.EquallySpacedRectSide\",\"uuid\":\"c87fdfc5-e8df-459e-b997-08543d0df41e\"},{\"content\":{\"connectorIds\":[\"Out1\",\"Out2\"],\"side\":\"RIGHT\"},\"type\":\"ConnectorPlacement.EquallySpacedRectSide\",\"uuid\":\"2c60bf56-1d16-41c9-95da-6f31ce1e2453\"},{\"content\":{\"side\":\"TOP\"},\"type\":\"ConnectorPlacement.EquallySpacedRectSide\",\"uuid\":\"3204d3ae-6da8-4da9-829b-7d815393aaef\"}]},\"type\":\"ConnectorPlacement.EquallySpacedConnector\",\"uuid\":\"82e413f9-6f35-4bf6-9ebc-f322256f270e\"}],\"packageUris\":[\"http://schema.mathworks.com/mf0/Connector/R2020b\"],\"version\":\"1.0\"}"
  Bus Element Out1 : Outport  PortName=Enter System
  wires:
  Phone Call / Message Verfication Interface/1(Verified Though Phone Call / Message) -> Adapter/1(Verified Though Phone Call / Message)
  Two-Factor Authentication Interface/1(Select Phone Call) -> Phone Call / Message Verfication Interface/1(Select Phone Call)
  Two-Factor Authentication Interface/2(Select Email) -> Email Verification Interface/1(Select Email)
  Email Verification Interface/1(Verified Though Email) -> Adapter/2(Verified Though Email)
  Adapter/1(Enter System) -> Bus Element Out1/1
  Bus Element In1/1 -> Two-Factor Authentication Interface/1(Authenticate)

== system Online_Ordering_System_Component_Architecture/Account Management System/Customer Setting Interface ==
  Bus Element In1 : Inport  PortName=Login As Customer
  Bus Element Out1 : Outport  PortName=Customer

== system Online_Ordering_System_Component_Architecture/Account Management System/Merchant Setting Interface ==
  Bus Element In1 : Inport  PortName=Login As Merchant
  Bus Element Out2 : Outport  PortName=Merchant
  Bus Element Out1 : Outport  Port=2  PortName=Product Information Edit

== system Online_Ordering_System_Component_Architecture/Account Management System/New Customer Account Creation Interface ==
  Bus Element In1 : Inport  PortName=Making Account
  Bus Element Out1 : Outport  PortName=Login As Customer

== system Online_Ordering_System_Component_Architecture/Account Management System/New Merchant Account Creation Interface ==
  Bus Element In1 : Inport  PortName=Making Account
  Bus Element Out1 : Outport  PortName=Login As Merchant

== system Online_Ordering_System_Component_Architecture/Customer Support System /Feedback Interface ==
  Bus Element In1 : Inport  PortName=Running Server

== system Online_Ordering_System_Component_Architecture/Customer Support System /Live Chat Interface ==
  Bus Element In1 : Inport  PortName=Running Server

== system Online_Ordering_System_Component_Architecture/Customer Support System /Membership Interface ==
  Bus Element In1 : Inport  PortName=Running Server

== system Online_Ordering_System_Component_Architecture/Customer Support System /Subscription Service Interface ==
  Bus Element In1 : Inport  PortName=Running Server

== system Online_Ordering_System_Component_Architecture/Delivery System/Delivery Information Interface ==
  Bus Element In1 : Inport  PortName=Access GPS Features
  Bus Element In2 : Inport  Port=2  PortName=Running Server
  Bus Element Out1 : Outport  PortName=Delivery Process

== system Online_Ordering_System_Component_Architecture/Delivery System/GPS Tracking System ==
  Bus Element In1 : Inport  PortName=Delivery Process
  Bus Element In2 : Inport  Port=2  PortName=Running Server

== system Online_Ordering_System_Component_Architecture/Multi-Platform Compatible Operating System /Desktop Device Platform ==
  Bus Element In3 : Inport  PortName=Data Share From Mobile Devices
  Bus Element In2 : Inport  Port=2  PortName=Running Server
  Bus Element Out2 : Outport  PortName=Data Share From PC / Laptop

== system Online_Ordering_System_Component_Architecture/Multi-Platform Compatible Operating System /Mobile Device Platform ==
  Bus Element In2 : Inport  PortName=Running Server
  Bus Element In1 : Inport  Port=2  PortName=Data Share From PC / Laptop
  Bus Element Out1 : Outport  PortName=Data Share From Mobile Devices

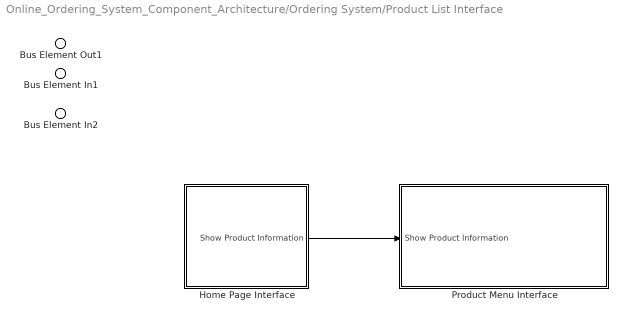
== system Online_Ordering_System_Component_Architecture/Ordering System/Product List Interface ==
  Bus Element In1 : Inport  PortName=Enter System
  Bus Element In2 : Inport  Port=2  PortName=Running Server
  Home Page Interface : Subsystem
      settings: PortSchema="{\"entries\":[{\"content\":{\"headerSize\":26,\"margin\":15,\"minimumSpacing\":25,\"sides\":[{\"content\":{},\"type\":\"ConnectorPlacement.EquallySpacedRectSide\",\"uuid\":\"d2ebed04-42f4-4bd6-aa56-c214d37abe86\"},{\"content\":{\"connectorIds\":[\"Out1\"],\"side\":\"RIGHT\"},\"type\":\"ConnectorPlacement.EquallySpacedRectSide\",\"uuid\":\"0a328130-2da5-4535-b8fd-dee261bd04a3\"},{\"content\":{\"side\":\"TOP\"},\"type\":\"ConnectorPlacement.EquallySpacedRectSide\",\"uuid\":\"410ea5eb-e20b-4523-bb7e-a86253749ceb\"}]},\"type\":\"ConnectorPlacement.EquallySpacedConnector\",\"uuid\":\"5600d62f-d466-4629-981b-50f24b9b11a3\"}],\"packageUris\":[\"http://schema.mathworks.com/mf0/Connector/R2020b\"],\"version\":\"1.0\"}"
  Product Menu Interface : Subsystem
      settings: PortSchema="{\"entries\":[{\"content\":{\"headerSize\":26,\"margin\":15,\"minimumSpacing\":25,\"sides\":[{\"content\":{\"connectorIds\":[\"In1\"]},\"type\":\"ConnectorPlacement.EquallySpacedRectSide\",\"uuid\":\"d2ebed04-42f4-4bd6-aa56-c214d37abe86\"},{\"content\":{\"side\":\"RIGHT\"},\"type\":\"ConnectorPlacement.EquallySpacedRectSide\",\"uuid\":\"0a328130-2da5-4535-b8fd-dee261bd04a3\"},{\"content\":{\"side\":\"TOP\"},\"type\":\"ConnectorPlacement.EquallySpacedRectSide\",\"uuid\":\"410ea5eb-e20b-4523-bb7e-a86253749ceb\"}]},\"type\":\"ConnectorPlacement.EquallySpacedConnector\",\"uuid\":\"5600d62f-d466-4629-981b-50f24b9b11a3\"}],\"packageUris\":[\"http://schema.mathworks.com/mf0/Connector/R2020b\"],\"version\":\"1.0\"}"
  Bus Element Out1 : Outport  PortName=Add To / Remove From / Clear Cart
  wires:
  Home Page Interface/1(Show Product Information) -> Product Menu Interface/1(Show Product Information)

== system Online_Ordering_System_Component_Architecture/Payment Management System / Gift Card // Coupons Payment Interface ==
  Bus Element In1 : Inport  PortName=Checkout
  Bus Element In2 : Inport  Port=2  PortName=Running Server
  Bus Element Out1 : Outport  PortName=Gift Card Payment

== system Online_Ordering_System_Component_Architecture/Payment Management System /Adapter ==
  In Bus Element : Inport  PortName=Online Payment
  Bus Element In2 : Inport  Port=2  PortName=Gift Card Payment
  Out Bus Element : Outport  PortName=Payment Valid
  wires:
  In Bus Element/1 -> Out Bus Element/1

== system Online_Ordering_System_Component_Architecture/Payment Management System /Online Payment Interface ==
  Bus Element In1 : Inport  PortName=Checkout
  Bus Element In2 : Inport  Port=2  PortName=Running Server
  Bus Element Out1 : Outport  PortName=Online Payment

== system Online_Ordering_System_Component_Architecture/Payment Management System /Payment Confirm Interface ==
  Bus Element In1 : Inport  PortName=Payment Valid
  Bus Element Out2 : Outport  PortName=Review Order

== system Online_Ordering_System_Component_Architecture/Payment Management System /Review Order Interface ==
  Bus Element In1 : Inport  PortName=Review Order
  Bus Element Out1 : Outport  PortName=Access GPS Feature

== system Online_Ordering_System_Component_Architecture/Product Management System/Product Availability Information ==
  Bus Element In1 : Inport  PortName=Check Availability
  Bus Element Out1 : Outport  PortName=Update Inventory Information

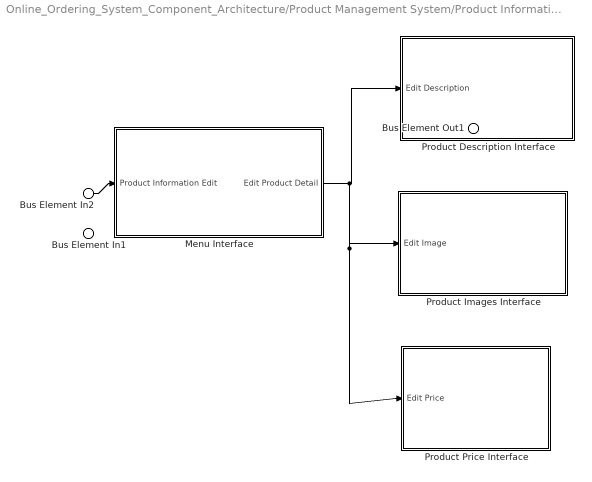
== system Online_Ordering_System_Component_Architecture/Product Management System/Product Information ==
  Bus Element In2 : Inport  PortName=Product Information Edit
  Bus Element In1 : Inport  Port=2  PortName=Running Server
  Menu Interface : Subsystem
      settings: PortSchema="{\"entries\":[{\"content\":{\"headerSize\":26,\"margin\":15,\"minimumSpacing\":25,\"sides\":[{\"content\":{\"connectorIds\":[\"In1\"]},\"type\":\"ConnectorPlacement.EquallySpacedRectSide\",\"uuid\":\"d2ebed04-42f4-4bd6-aa56-c214d37abe86\"},{\"content\":{\"connectorIds\":[\"Out1\"],\"side\":\"RIGHT\"},\"type\":\"ConnectorPlacement.EquallySpacedRectSide\",\"uuid\":\"0a328130-2da5-4535-b8fd-dee261bd04a3\"},{\"content\":{\"side\":\"TOP\"},\"type\":\"ConnectorPlacement.EquallySpacedRectSide\",\"uuid\":\"410ea5eb-e20b-4523-bb7e-a86253749ceb\"}]},\"type\":\"ConnectorPlacement.EquallySpacedConnector\",\"uuid\":\"5600d62f-d466-4629-981b-50f24b9b11a3\"}],\"packageUris\":[\"http://schema.mathworks.com/mf0/Connector/R2020b\"],\"version\":\"1.0\"}"
  Product Description Interface : Subsystem
      settings: PortSchema="{\"entries\":[{\"content\":{\"headerSize\":26,\"margin\":15,\"minimumSpacing\":25,\"sides\":[{\"content\":{\"connectorIds\":[\"In1\"]},\"type\":\"ConnectorPlacement.EquallySpacedRectSide\",\"uuid\":\"c87fdfc5-e8df-459e-b997-08543d0df41e\"},{\"content\":{\"side\":\"RIGHT\"},\"type\":\"ConnectorPlacement.EquallySpacedRectSide\",\"uuid\":\"2c60bf56-1d16-41c9-95da-6f31ce1e2453\"},{\"content\":{\"side\":\"TOP\"},\"type\":\"ConnectorPlacement.EquallySpacedRectSide\",\"uuid\":\"3204d3ae-6da8-4da9-829b-7d815393aaef\"}]},\"type\":\"ConnectorPlacement.EquallySpacedConnector\",\"uuid\":\"82e413f9-6f35-4bf6-9ebc-f322256f270e\"}],\"packageUris\":[\"http://schema.mathworks.com/mf0/Connector/R2020b\"],\"version\":\"1.0\"}"
  Product Images Interface : Subsystem
      settings: PortSchema="{\"entries\":[{\"content\":{\"headerSize\":26,\"margin\":15,\"minimumSpacing\":25,\"sides\":[{\"content\":{\"connectorIds\":[\"In1\"]},\"type\":\"ConnectorPlacement.EquallySpacedRectSide\",\"uuid\":\"c87fdfc5-e8df-459e-b997-08543d0df41e\"},{\"content\":{\"side\":\"RIGHT\"},\"type\":\"ConnectorPlacement.EquallySpacedRectSide\",\"uuid\":\"2c60bf56-1d16-41c9-95da-6f31ce1e2453\"},{\"content\":{\"side\":\"TOP\"},\"type\":\"ConnectorPlacement.EquallySpacedRectSide\",\"uuid\":\"3204d3ae-6da8-4da9-829b-7d815393aaef\"}]},\"type\":\"ConnectorPlacement.EquallySpacedConnector\",\"uuid\":\"82e413f9-6f35-4bf6-9ebc-f322256f270e\"}],\"packageUris\":[\"http://schema.mathworks.com/mf0/Connector/R2020b\"],\"version\":\"1.0\"}"
  Product Price Interface : Subsystem
      settings: PortSchema="{\"entries\":[{\"content\":{\"headerSize\":26,\"margin\":15,\"minimumSpacing\":25,\"sides\":[{\"content\":{\"connectorIds\":[\"In1\"]},\"type\":\"ConnectorPlacement.EquallySpacedRectSide\",\"uuid\":\"c87fdfc5-e8df-459e-b997-08543d0df41e\"},{\"content\":{\"side\":\"RIGHT\"},\"type\":\"ConnectorPlacement.EquallySpacedRectSide\",\"uuid\":\"2c60bf56-1d16-41c9-95da-6f31ce1e2453\"},{\"content\":{\"side\":\"TOP\"},\"type\":\"ConnectorPlacement.EquallySpacedRectSide\",\"uuid\":\"3204d3ae-6da8-4da9-829b-7d815393aaef\"}]},\"type\":\"ConnectorPlacement.EquallySpacedConnector\",\"uuid\":\"82e413f9-6f35-4bf6-9ebc-f322256f270e\"}],\"packageUris\":[\"http://schema.mathworks.com/mf0/Connector/R2020b\"],\"version\":\"1.0\"}"
  Bus Element Out1 : Outport  PortName=Check Availability
  wires:
  Bus Element In2/1 -> Menu Interface/1(Product Information Edit)
  Menu Interface/1(Edit Product Detail) -> Product Price Interface/1(Edit Price), Product Images Interface/1(Edit Image), Product Description Interface/1(Edit Description)

== system Online_Ordering_System_Component_Architecture/Product Management System/Updated Inventory ==
  Bus Element In1 : Inport  PortName=Update Inventory Information

== system Online_Ordering_System_Component_Architecture/Account Management System/Authentication System /Adapter ==
  Bus Element In1 : Inport  PortName=Verified Though Phone Call / Message
  In Bus Element : Inport  Port=2  PortName=Verified Though Email
  Out Bus Element : Outport  PortName=Enter System
  wires:
  In Bus Element/1 -> Out Bus Element/1

== system Online_Ordering_System_Component_Architecture/Account Management System/Authentication System /Email Verification Interface ==
  Bus Element In1 : Inport  PortName=Select Email
  Bus Element Out1 : Outport  PortName=Verified Though Email

== system Online_Ordering_System_Component_Architecture/Account Management System/Authentication System /Phone Call // Message Verfication Interface ==
  Bus Element In1 : Inport  PortName=Select Phone Call
  Bus Element Out1 : Outport  PortName=Verified Though Phone Call / Message

== system Online_Ordering_System_Component_Architecture/Account Management System/Authentication System /Two-Factor Authentication Interface ==
  Bus Element In1 : Inport  PortName=Authenticate
  Bus Element Out1 : Outport  PortName=Select Phone Call
  Bus Element Out2 : Outport  Port=2  PortName=Select Email

== system Online_Ordering_System_Component_Architecture/Ordering System/Product List Interface/Home Page Interface ==
  Bus Element Out1 : Outport  PortName=Show Product Information
